simulink library "lib_controller"  (R2015a)
settings: Solver=ode45  StartTime=0.0  StopTime=10.0  RelTol=1e-3
values from neighbouring files (symbols this model uses):
  CG_0 = [0,0,0.02]'    [SetupComplete.m]
  g = 9.81    [SetupComplete.m]
  h_M = 0.064    [SetupComplete.m]
  I_BAC_0 = [ Ix,0,Ixz;0,Iy,0;Ixz,0,Iz]    [SetupComplete.m]
  l = 0.3450    (= 0.345)    [NDI_components.m]    (also in SetupComplete.m; robust_controller.m)
  m = 3.51    [SetupComplete.m]
  m_0 = 2.61    [SetupComplete.m]
  m_M = 0.300    (= 0.3)    [SetupComplete.m]
  T_sim = 0.01    [Run3Copter.m]
undefined symbols (not defined in the file or in its folder): Theta_1_roll_last, Theta_2_roll_last, Theta_3_roll_last, V_long_lastA_w_z, V_long_lastAoA, V_roll_last, V_yaw_last, W_long_lastA_w_z, W_long_lastAoA, W_roll_last, W_yaw_last
libraries: simulink x65, Adaptive_FaultTolerantControl x8, lib_controller x5, qcatlib x4, dspinverses x4, aerolibtransform2 x3, aerolib6dofsys x1
(part 3 of 10)

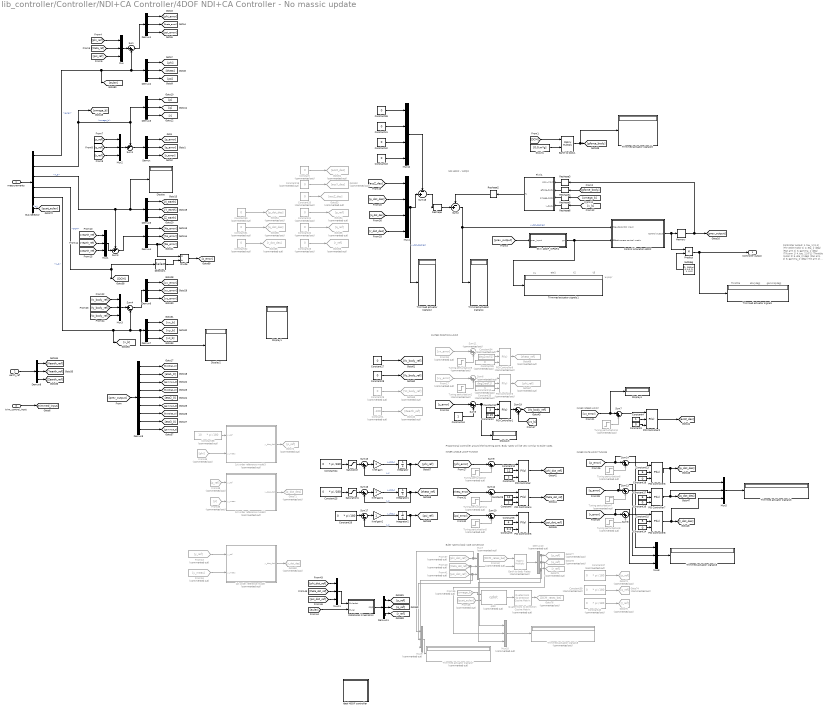
== system lib_controller/Controller/NDI+CA Controller/4DOF NDI+CA Controller - No massic update ==
  note: w
      | p
      | q
      | r
  note: t1
  note: t2
  note: t3
  note: eta1
  note: OUTER POSITION LOOP
  note: gamma[deg]
  note: eta [deg]
  note: Throttle
  note: Controller output:
      | 1. tau_1 [0-1] (Thr ottle motor 1)
      | 2. eta_1 (deg)  (Pan arm 1)
      | 3. gamma_1 (deg)  (Tilt arm 1)
      |
      | 4. tau_2 [0-1] (Throttle motor 2)
      | 5. eta_2 (deg)  (Pan arm 2)
      | 6. gamma_2 (deg)  (Tilt arm 2)
      |
      | 7. tau_3 [0-1] (Throttle motor 3)
      | 8. eta_3 (deg)  (Pan arm  3)
      | 9. gamma_3 (deg)  (Tilt arm 3)
  note: Proportional controller around the hovering point. Body rates will be very similar to euler rates.
  note: INNER RATE LOOP TUNING
  note: INNER ANGLE LOOP TUNING
  note: INNER SPEED LOOP
  note: NDI 4DOF - WPQR
  note: Euler rate to body rate conversion
  measurements : Inport
  earth_ref : Inport  Port=2
  trim_control_input : Inport  Port=3
  1st order reference model : Subsystem  Commented=on  mask(1st order model reference block){Kref=1, Kb=20, fi=0.25, fc=0.5, Kf=1}
      mask prompts: Kref "1st order reference gain"; Kb "Bandwidth gain"; fi "Integral gain"; fc "Command FF gain"; Kf "Command_dot FF gain"
      mask help:
      | Generates a desired first order derivative of a commanded output taking
      | into account the current measured output.
      | Kref is the gain that determines the first order system between y_ref and
      | y_commanded signals. Ycom/Yref = Kref/(1 + Kref)
      | fi and fc can be defaulted to 0.25 and 0.5 for a critically damped 2nd
      | order response between y_meas and the error signal (y_com - y_meas) considering
      | a perfect dynamic inversion.
      mask Help:
      | Juan Herrero Macias <jn.herrerom@gmail.com>
      | This architecture can be found and explained in Fault-tolerant Flight
      | Control and Guidance Systems, Ducard, Guillaume.
      mask TypeOptions Kref: Kref gain/Gain
      mask TypeOptions Kb: Bandwidth gain/Gain
      mask TypeOptions fi: Integral gain/Gain
      mask TypeOptions fc: Command FF gain/Gain
      mask TypeOptions Kf: Command_dot FF gain/Gain
  1st order reference model2 : Subsystem  Commented=on  mask(1st order model reference block){Kref=2, Kb=2, fi=0.25, fc=0.5, Kf=1}
      mask prompts: Kref "1st order reference gain"; Kb "Bandwidth gain"; fi "Integral gain"; fc "Command FF gain"; Kf "Command_dot FF gain"
      mask help:
      | Generates a desired first order derivative of a commanded output taking
      | into account the current measured output.
      | Kref is the gain that determines the first order system between y_ref and
      | y_commanded signals. Ycom/Yref = Kref/(1 + Kref)
      | fi and fc can be defaulted to 0.25 and 0.5 for a critically damped 2nd
      | order response between y_meas and the error signal (y_com - y_meas) considering
      | a perfect dynamic inversion.
      mask Help:
      | Juan Herrero Macias <jn.herrerom@gmail.com>
      | This architecture can be found and explained in Fault-tolerant Flight
      | Control and Guidance Systems, Ducard, Guillaume.
      mask TypeOptions Kref: Kref gain/Gain
      mask TypeOptions Kb: Bandwidth gain/Gain
      mask TypeOptions fi: Integral gain/Gain
      mask TypeOptions fc: Command FF gain/Gain
      mask TypeOptions Kf: Command_dot FF gain/Gain
  1st order reference model3 : Subsystem  Commented=on  mask(1st order model reference block){Kref=2, Kb=2, fi=0.25, fc=0, Kf=0}
      mask prompts: Kref "1st order reference gain"; Kb "Bandwidth gain"; fi "Integral gain"; fc "Command FF gain"; Kf "Command_dot FF gain"
      mask help:
      | Generates a desired first order derivative of a commanded output taking
      | into account the current measured output.
      | Kref is the gain that determines the first order system between y_ref and
      | y_commanded signals. Ycom/Yref = Kref/(1 + Kref)
      | fi and fc can be defaulted to 0.25 and 0.5 for a critically damped 2nd
      | order response between y_meas and the error signal (y_com - y_meas) considering
      | a perfect dynamic inversion.
      mask Help:
      | Juan Herrero Macias <jn.herrerom@gmail.com>
      | This architecture can be found and explained in Fault-tolerant Flight
      | Control and Guidance Systems, Ducard, Guillaume.
      mask TypeOptions Kref: Kref gain/Gain
      mask TypeOptions Kb: Bandwidth gain/Gain
      mask TypeOptions fi: Integral gain/Gain
      mask TypeOptions fc: Command FF gain/Gain
      mask TypeOptions Kf: Command_dot FF gain/Gain
  Bus Selector : BusSelector  OutputSignals=euler,omega_b,X_e,DCM,V_b,q
  Constant{,19..23,29..33,35} (12 alike) : Constant  Commented=on  Value=0
  Constant1 : Constant  Commented=on  Value=-100
  Constant10 : Constant  Value=12
  Constant11 : Constant  Value=3
  Constant12 : Constant  Commented=on  Value=deg2rad(1)
  Constant13 : Constant  Value=6
  Constant{3,14,16,18,27..28,36,41..43} (10 alike) : Constant  Value=0
  Constant15 : Constant  Value=5
  Constant17 : Constant  Value=6
  Constant2 : Constant  Value=0.15
  Constant24 : Constant  Value="0     * pi /180"
  Constant25 : Constant  Value="0     * pi /180"
  Constant26 : Constant  Value="0     * pi /180"
  Constant34 : Constant  Commented=on  Value=deg2rad(1)
  Constant37 : Constant  Commented=on  Value="0     * pi /180"
  Constant38 : Constant  Commented=on  Value="10     * pi /180"
  Constant39 : Constant  Commented=on  Value="0     * pi /180"
  Constant4 : Constant
  Constant40 : Constant  Commented=on  Value="0     * pi /180"
  Constant44 : Constant
  Constant5 : Constant  Value=0.4
  Constant6 : Constant  Value=4
  Constant7 : Constant  Value=3
  Constant8 : Constant  Value=12
  Constant9 : Constant  Value=3
  Control Allocation 4DOF : Subsystem  Variant=on  OverrideUsingVariant=(default)
  Demux{,1..8,11} (10 alike) : Demux  Outputs=3
  Demux10 : Demux  Commented=on  Outputs=3
  Demux9 : Demux  Outputs=9
  Display{,1..4} (5 alike) : Display
  Divide : Product  Inputs=*/
  Earth to body Rates : Product  Commented=on  Multiplication=Matrix(*)
  Earth to body1 : Product  Multiplication=Matrix(*)
  F(X)1 : MATLAB Function  TreatAsAtomicUnit=on
  From13 : From  Commented=on  GotoTag=y_ref
  From17 : From  Commented=on  GotoTag=vy_error
  From18 : From  Commented=on  GotoTag=vx_error
  From25 : From  Commented=on  GotoTag=quat_euler
  From34 : From  Commented=on  GotoTag=y_meas
  From35 : From  Commented=on  GotoTag=phi
  From36 : From  Commented=on  GotoTag=omega_b
  From37 : From  Commented=on  GotoTag=phi_dot_ref
  From38 : From  Commented=on  GotoTag=p_ref
  From39 : From  Commented=on  GotoTag=p
  From40 : From  Commented=on  GotoTag=theta_dot_ref
  From41 : From  Commented=on  GotoTag=psi_dot_ref
  From42 : From  Commented=on  GotoTag=DCM_rates_be
  G(X) 4DOF_WPQR1 : MATLAB Function  TreatAsAtomicUnit=on
  Goto40 : Goto  Commented=on  GotoTag=Zearth_ref
  Goto51 : Goto  Commented=on  GotoTag=accX_des
  Goto52 : Goto  Commented=on  GotoTag=accY_des
  Goto53 : Goto  Commented=on  GotoTag=accZ_des
  Goto{54,72..73,77} (4 alike) : Goto  Commented=on  GotoTag=p_ref
  Goto55 : Goto  Commented=on  GotoTag=q_ref
  Goto56 : Goto  Commented=on  GotoTag=r_ref
  Goto60 : Goto  Commented=on  GotoTag=y_dot_des
  Goto63 : Goto  Commented=on  GotoTag=Vz_body_ref
  Goto64 : Goto  Commented=on  GotoTag=p_dot_des
  Goto65 : Goto  Commented=on  GotoTag=q_dot_des
  Goto66 : Goto  Commented=on  GotoTag=r_dot_des
  Goto67 : Goto  Commented=on  GotoTag=phi_ref
  Goto68 : Goto  Commented=on  GotoTag=theta_ref
  Goto71 : Goto  Commented=on  GotoTag=p_dot_des
  Goto74 : Goto  Commented=on  GotoTag=q_ref
  Goto75 : Goto  Commented=on  GotoTag=r_ref
  Goto76 : Goto  Commented=on  GotoTag=DCM_rates_be
  Goto78 : Goto  Commented=on  GotoTag=q_ref
  Goto79 : Goto  Commented=on  GotoTag=r_ref
  Gravity : Constant  Value=[0;0;m*g]
  Ideal 4DOF controller : Subsystem
  Integrator : Integrator
  Integrator1 : Integrator
  Integrator2 : Integrator
  Kref gain : Gain
  Kref gain1 : Gain
  Kref gain2 : Gain
  Memory : Memory  X0=[0,0,0,0,0,0,0,0,0]  LinearizeAsDelay=on
  Mux{,1..3,5,8,11} (7 alike) : Mux  Inputs=3
  Mux10 : Mux  Commented=on  Inputs=3
  Mux12 : Mux
  Mux4 : Mux
  Mux7 : Mux  Commented=on  Inputs=3
  Mux9 : Mux  Commented=on  Inputs=3
  PID Controller{,1..2,4..5,8} (6 alike) : simulink/Continuous/PID Controller  Controller=PI  TimeDomain=Continuous-time  SampleTime=-1  IntegratorMethod=Forward Euler  FilterMethod=Forward Euler  Form=Parallel  UseFilter=on  ControllerParametersSource=external  P=1  I=1  D=0  N=100  InitialConditionSource=internal  InitialConditionForIntegrator=0  InitialConditionForFilter=0  ExternalReset=none  LimitOutput=off  UpperSaturationLimit=inf  LowerSaturationLimit=-inf  LinearizeAsGain=on  AntiWindupMode=none  Kb=1  TrackingMode=off  Kt=1  PParamMin=[]  PParamMax=[]  IParamMin=[]  IParamMax=[]  DParamMin=[]  DParamMax=[]  NParamMin=[]  NParamMax=[]  KbParamMin=[]  KbParamMax=[]  KtParamMin=[]  KtParamMax=[]  POutMin=[]  POutMax=[]  IOutMin=[]  IOutMax=[]  DOutMin=[]  DOutMax=[]  NOutMin=[]  NOutMax=[]  KbOutMin=[]  KbOutMax=[]  KtOutMin=[]  KtOutMax=[]  IntegratorOutMin=[]  IntegratorOutMax=[]  FilterOutMin=[]  FilterOutMax=[]  SumOutMin=[]  SumOutMax=[]  SumI1OutMin=[]  SumI1OutMax=[]  SumI2OutMin=[]  SumI2OutMax=[]  SumI3OutMin=[]  SumI3OutMax=[]  SumDOutMin=[]  SumDOutMax=[]  SaturationOutMin=[]  SaturationOutMax=[]  IntegratorContinuousStateAttributes=''  IntegratorStateMustResolveToSignalObject=off  IntegratorRTWStateStorageClass=Auto  FilterContinuousStateAttributes=''  FilterStateMustResolveToSignalObject=off  FilterRTWStateStorageClass=Auto  DifferentiatorICPrevScaledInput=0  DifferentiatorOutMin=[]  DifferentiatorOutMax=[]
  PID Controller3 : simulink/Continuous/PID Controller  Commented=on  Controller=PI  TimeDomain=Continuous-time  SampleTime=-1  IntegratorMethod=Forward Euler  FilterMethod=Forward Euler  Form=Parallel  UseFilter=on  ControllerParametersSource=external  P=1  I=1  D=0  N=100  InitialConditionSource=internal  InitialConditionForIntegrator=0  InitialConditionForFilter=0  ExternalReset=none  LimitOutput=off  UpperSaturationLimit=inf  LowerSaturationLimit=-inf  LinearizeAsGain=on  AntiWindupMode=none  Kb=1  TrackingMode=off  Kt=1  PParamMin=[]  PParamMax=[]  IParamMin=[]  IParamMax=[]  DParamMin=[]  DParamMax=[]  NParamMin=[]  NParamMax=[]  KbParamMin=[]  KbParamMax=[]  KtParamMin=[]  KtParamMax=[]  POutMin=[]  POutMax=[]  IOutMin=[]  IOutMax=[]  DOutMin=[]  DOutMax=[]  NOutMin=[]  NOutMax=[]  KbOutMin=[]  KbOutMax=[]  KtOutMin=[]  KtOutMax=[]  IntegratorOutMin=[]  IntegratorOutMax=[]  FilterOutMin=[]  FilterOutMax=[]  SumOutMin=[]  SumOutMax=[]  SumI1OutMin=[]  SumI1OutMax=[]  SumI2OutMin=[]  SumI2OutMax=[]  SumI3OutMin=[]  SumI3OutMax=[]  SumDOutMin=[]  SumDOutMax=[]  SaturationOutMin=[]  SaturationOutMax=[]  IntegratorContinuousStateAttributes=''  IntegratorStateMustResolveToSignalObject=off  IntegratorRTWStateStorageClass=Auto  FilterContinuousStateAttributes=''  FilterStateMustResolveToSignalObject=off  FilterRTWStateStorageClass=Auto  DifferentiatorICPrevScaledInput=0  DifferentiatorOutMin=[]  DifferentiatorOutMax=[]
  PID Controller6 : simulink/Continuous/PID Controller  Controller=PI  TimeDomain=Continuous-time  SampleTime=-1  IntegratorMethod=Forward Euler  FilterMethod=Forward Euler  Form=Parallel  UseFilter=on  ControllerParametersSource=external  P=121.80671459326  I=327.532586687046  D=0  N=100  InitialConditionSource=internal  InitialConditionForIntegrator=0  InitialConditionForFilter=0  ExternalReset=none  LimitOutput=off  UpperSaturationLimit=inf  LowerSaturationLimit=-inf  LinearizeAsGain=on  AntiWindupMode=none  Kb=1  TrackingMode=off  Kt=1  PParamMin=[]  PParamMax=[]  IParamMin=[]  IParamMax=[]  DParamMin=[]  DParamMax=[]  NParamMin=[]  NParamMax=[]  KbParamMin=[]  KbParamMax=[]  KtParamMin=[]  KtParamMax=[]  POutMin=[]  POutMax=[]  IOutMin=[]  IOutMax=[]  DOutMin=[]  DOutMax=[]  NOutMin=[]  NOutMax=[]  KbOutMin=[]  KbOutMax=[]  KtOutMin=[]  KtOutMax=[]  IntegratorOutMin=[]  IntegratorOutMax=[]  FilterOutMin=[]  FilterOutMax=[]  SumOutMin=[]  SumOutMax=[]  SumI1OutMin=[]  SumI1OutMax=[]  SumI2OutMin=[]  SumI2OutMax=[]  SumI3OutMin=[]  SumI3OutMax=[]  SumDOutMin=[]  SumDOutMax=[]  SaturationOutMin=[]  SaturationOutMax=[]  IntegratorContinuousStateAttributes=''  IntegratorStateMustResolveToSignalObject=off  IntegratorRTWStateStorageClass=Auto  FilterContinuousStateAttributes=''  FilterStateMustResolveToSignalObject=off  FilterRTWStateStorageClass=Auto  DifferentiatorICPrevScaledInput=0  DifferentiatorOutMin=[]  DifferentiatorOutMax=[]
  PID Controller7 : simulink/Continuous/PID Controller  Controller=PI  TimeDomain=Continuous-time  SampleTime=-1  IntegratorMethod=Forward Euler  FilterMethod=Forward Euler  Form=Parallel  UseFilter=on  ControllerParametersSource=external  P=244.169484479421  I=1759.80724182952  D=0  N=100  InitialConditionSource=internal  InitialConditionForIntegrator=0  InitialConditionForFilter=0  ExternalReset=none  LimitOutput=off  UpperSaturationLimit=inf  LowerSaturationLimit=-inf  LinearizeAsGain=on  AntiWindupMode=none  Kb=1  TrackingMode=off  Kt=1  PParamMin=[]  PParamMax=[]  IParamMin=[]  IParamMax=[]  DParamMin=[]  DParamMax=[]  NParamMin=[]  NParamMax=[]  KbParamMin=[]  KbParamMax=[]  KtParamMin=[]  KtParamMax=[]  POutMin=[]  POutMax=[]  IOutMin=[]  IOutMax=[]  DOutMin=[]  DOutMax=[]  NOutMin=[]  NOutMax=[]  KbOutMin=[]  KbOutMax=[]  KtOutMin=[]  KtOutMax=[]  IntegratorOutMin=[]  IntegratorOutMax=[]  FilterOutMin=[]  FilterOutMax=[]  SumOutMin=[]  SumOutMax=[]  SumI1OutMin=[]  SumI1OutMax=[]  SumI2OutMin=[]  SumI2OutMax=[]  SumI3OutMin=[]  SumI3OutMax=[]  SumDOutMin=[]  SumDOutMax=[]  SaturationOutMin=[]  SaturationOutMax=[]  IntegratorContinuousStateAttributes=''  IntegratorStateMustResolveToSignalObject=off  IntegratorRTWStateStorageClass=Auto  FilterContinuousStateAttributes=''  FilterStateMustResolveToSignalObject=off  FilterRTWStateStorageClass=Auto  DifferentiatorICPrevScaledInput=0  DifferentiatorOutMin=[]  DifferentiatorOutMax=[]
  PID Controller9 : simulink/Continuous/PID Controller  Commented=on  Controller=PI  TimeDomain=Continuous-time  SampleTime=-1  IntegratorMethod=Forward Euler  FilterMethod=Forward Euler  Form=Parallel  UseFilter=on  ControllerParametersSource=external  P=1  I=1  D=0  N=100  InitialConditionSource=internal  InitialConditionForIntegrator=0  InitialConditionForFilter=0  ExternalReset=none  LimitOutput=off  UpperSaturationLimit=inf  LowerSaturationLimit=-inf  LinearizeAsGain=on  AntiWindupMode=none  Kb=1  TrackingMode=off  Kt=1  PParamMin=[]  PParamMax=[]  IParamMin=[]  IParamMax=[]  DParamMin=[]  DParamMax=[]  NParamMin=[]  NParamMax=[]  KbParamMin=[]  KbParamMax=[]  KtParamMin=[]  KtParamMax=[]  POutMin=[]  POutMax=[]  IOutMin=[]  IOutMax=[]  DOutMin=[]  DOutMax=[]  NOutMin=[]  NOutMax=[]  KbOutMin=[]  KbOutMax=[]  KtOutMin=[]  KtOutMax=[]  IntegratorOutMin=[]  IntegratorOutMax=[]  FilterOutMin=[]  FilterOutMax=[]  SumOutMin=[]  SumOutMax=[]  SumI1OutMin=[]  SumI1OutMax=[]  SumI2OutMin=[]  SumI2OutMax=[]  SumI3OutMin=[]  SumI3OutMax=[]  SumDOutMin=[]  SumDOutMax=[]  SaturationOutMin=[]  SaturationOutMax=[]  IntegratorContinuousStateAttributes=''  IntegratorStateMustResolveToSignalObject=off  IntegratorRTWStateStorageClass=Auto  FilterContinuousStateAttributes=''  FilterStateMustResolveToSignalObject=off  FilterRTWStateStorageClass=Auto  DifferentiatorICPrevScaledInput=0  DifferentiatorOutMin=[]  DifferentiatorOutMax=[]
  Product : Product
  Quaternions to Direction Cosine Matrix : aerolibtransform2/Quaternions to  Direction Cosine Matrix  Commented=on
  Reshape : Reshape  OutputDimensionality=Column vector (2-D)
  Reshape2 : Reshape  OutputDimensionality=Column vector (2-D)  OutputDimensions=[6,1]
  Reshape{3..6} (4 alike) : Reshape  OutputDimensions=[6,1]
  Rotational Kinematics : MATLAB Function  TreatAsAtomicUnit=on
  Saturation : Saturate  UpperLimit=30  LowerLimit=-30
  Saturation1 : Saturate  UpperLimit=30  LowerLimit=-30
  Selector1 : Selector  NumberOfDimensions=2  InputPortWidth=[9]  IndexOptions=Index vector (dialog),Index vector (dialog)  Indices=3,3  OutputSizes=1,1
  Sum{,4,15..17} (5 alike) : Sum  Inputs=|+-
  Sum{1..3,18} (4 alike) : Sum  Inputs=-+|
  Sum{5,7..10,12..14,19} (9 alike) : Sum  Inputs=|++
  Sum11 : Sum  Commented=on  Inputs=|++
  Sum6 : Sum  Commented=on  Inputs=|++
  Trimmed actuator signals{,1..6} (7 alike) : Display
  Trimmed actuator signals7 : Display  Commented=on
  Trimmed actuator signals8 : Display  Commented=on
  Tuning perturbation{,5..6,8} (4 alike) : Step  Commented=on  Time=20  After=3*pi/180  SampleTime=0
  Tuning perturbation2 : Step  Commented=on  Time=20  SampleTime=0
  Tuning perturbation3 : Step  Commented=on  Time=20  SampleTime=0
  Tuning perturbation4 : Step  Commented=on  Time=20  After=-3*pi/180  SampleTime=0
  Tuning perturbation7 : Step  Commented=on  Time=20  After=-3*pi/180  SampleTime=0
  Tuning perturbation9 : Step  Commented=on  Time=20  SampleTime=0
  qdot : aerolib6dofsys/DCM & Euler Angles (Quaternion)/qdot  Commented=on
  rad2deg : Constant  Value=[1, 180/pi, 0,1,0, 0, 1, 0,0]
  Controller output : Outport
  wires:
  [vz_b] -> Sum19/2
  Sum19/1 -> [Vz_body_ref]
  PID Controller1/1 -> Sum19/1
  Selector1/1 -> Divide/2
  Demux4/3 -> [Ze_error], Divide/1
  Saturation1/1 -> Sum16/1
  Saturation/1 -> Sum15/1
  Sum18/1 -> Reshape/1
  Mux12/1 -> Sum18/1
  Constant43/1 -> Mux12/4
  Constant42/1 -> Mux12/3
  Constant41/1 -> Mux12/2
  Constant36/1 -> Mux12/1
  Mux11/1 -> Rotational Kinematics/1(Eulerdot)
  [psi_dot_ref] -> Mux11/3
  [theta_dot_ref] -> Mux11/2
  [phi_dot_ref] -> Mux11/1
  Rotational Kinematics/1(PQR) -> Demux11/1
  Demux11/3 -> [r_ref]
  Demux11/2 -> [q_ref]
  Demux11/1 -> [p_ref]
  [euler] -> Rotational Kinematics/2(Euler)
  Mux10/1 -> Trimmed actuator signals8/1
  Demux10/3 -> Mux10/3, Goto79/1
  Demux10/2 -> Goto78/1, Mux10/2
  Demux10/1 -> Goto77/1, Mux10/1
  Mux9/1 -> Trimmed actuator signals7/1
  From41/1 -> Mux7/3, Mux9/3
  From40/1 -> Mux7/2, Mux9/2
  From37/1 -> Mux7/1, Mux9/1
  Quaternions to Direction Cosine Matrix/1 -> Goto76/1
  From25/1 -> qdot/2
  qdot/1 -> Quaternions to Direction Cosine Matrix/1
  From36/1 -> qdot/1
  Earth to body Rates/1 -> Demux10/1
  From42/1 -> Earth to body Rates/1
  Mux7/1 -> Earth to body Rates/2
  Bus Selector/6 -> [quat_euler]  "<q>"
  Divide/1 -> [z_error]
  Constant40/1 -> Goto75/1
  Constant39/1 -> Goto74/1
  Constant37/1 -> Goto73/1
  Constant14/1 -> PID Controller8/3
  Constant18/1 -> PID Controller6/3
  Sum17/1 -> Kref gain2/1
  Kref gain2/1 -> Integrator2/1  "y_dot_c"
  Integrator2/1 -> [psi_ref], Sum17/2  "y_c"
  Constant26/1 -> Sum17/1
  Sum16/1 -> Kref gain1/1
  Kref gain1/1 -> Integrator1/1  "y_dot_c"
  Integrator1/1 -> Sum16/2, [theta_ref]  "y_c"
  Constant25/1 -> Saturation1/1
  Sum15/1 -> Kref gain/1
  Kref gain/1 -> Integrator/1  "y_dot_c"
  Integrator/1 -> [phi_ref], Sum15/2  "y_c"
  Constant24/1 -> Saturation/1
  Constant38/1 -> 1st order reference model3/1(y_ref)
  1st order reference model3/1(y_des_dot) -> Goto72/1
  From35/1 -> 1st order reference model3/2(y_meas)
  From38/1 -> 1st order reference model2/1(y_ref)
  1st order reference model2/1(y_des_dot) -> Goto71/1
  From39/1 -> 1st order reference model2/2(y_meas)
  G(X) 4DOF_WPQR1/1(gx) -> Control Allocation 4DOF/2(Effectiveness control matrix), Trimmed actuator signals1/1
  PID Controller9/1 -> Goto68/1
  Tuning perturbation9/1 -> Sum11/2
  From18/1 -> Sum11/1
  Sum11/1 -> PID Controller9/1
  Constant35/1 -> PID Controller9/3
  Constant34/1 -> PID Controller9/2
  PID Controller3/1 -> Goto67/1
  Tuning perturbation2/1 -> Sum6/2
  From17/1 -> Sum6/1
  Sum6/1 -> PID Controller3/1
  Constant33/1 -> PID Controller3/3
  Constant12/1 -> PID Controller3/2
  Constant44/1 -> Sum5/2
  [z_error] -> Sum5/1
  Sum5/1 -> PID Controller1/1, Display3/1
  Constant2/1 -> PID Controller1/3
  Constant11/1 -> PID Controller1/2
  Constant1/1 -> Goto40/1
  [r_dot_des] -> Mux4/4
  [q_dot_des] -> Mux4/3
  [p_dot_des] -> Mux4/2
  [accZ_des] -> Mux4/1
  [prev_output] -> G(X) 4DOF_WPQR1/1(prev_input)
  Control Allocation 4DOF/1(Control output) -> Memory/1, Product/1
  Sum2/1 -> Control Allocation 4DOF/1(Pseudocontrol input), Trimmed actuator signals4/1  "y_dot_desired"
  Constant13/1 -> PID Controller6/2
  Sum3/1 -> Demux4/1
  Constant32/1 -> Goto66/1
  Constant31/1 -> Goto65/1
  Constant30/1 -> Goto64/1
  Memory/1 -> [prev_output], Reshape3/1
  [DCM] -> Earth to body1/1
  Mux8/1 -> Trimmed actuator signals5/1
  [r_error] -> Sum8/1, Mux8/3
  [q_error] -> Sum13/1, Mux8/2
  [p_error] -> Sum14/1, Mux8/1
  [psi_error] -> Sum10/1
  [theta_error] -> Sum12/1
  [phi_error] -> Sum9/1
  Constant29/1 -> Goto63/1
  Constant28/1 -> [Vy_body_ref]
  Constant27/1 -> [Vx_body_ref]
  PID Controller2/1 -> [accZ_des]
  Mux5/1 -> Trimmed actuator signals3/1
  1st order reference model/1(y_des_dot) -> Goto60/1
  From34/1 -> 1st order reference model/2(y_meas)
  From13/1 -> 1st order reference model/1(y_ref)
  rad2deg/1 -> Product/2
  Product/1 -> Controller output/1, Trimmed actuator signals/1
  Constant23/1 -> Goto56/1
  Constant22/1 -> Goto55/1
  Constant21/1 -> Goto54/1
  Constant20/1 -> Goto53/1
  Constant19/1 -> Goto52/1
  Constant/1 -> Goto51/1
  [v_b] -> Reshape6/1
  Reshape6/1 -> F(X)1/4(v_body)
  Reshape5/1 -> F(X)1/3(omega_body)
  Reshape4/1 -> F(X)1/2(gforce_body)
  [omega_b] -> Reshape5/1
  Reshape3/1 -> F(X)1/1(prev_input)
  Reshape2/1 -> Sum2/1
  Reshape/1 -> Sum2/2
  Mux4/1 -> Sum18/2, Trimmed actuator signals2/1  "y_dot_desired"
  Tuning perturbation7/1 -> Sum13/2
  Tuning perturbation6/1 -> Sum14/2
  Tuning perturbation8/1 -> Sum8/2
  Sum13/1 -> PID Controller7/1
  Sum8/1 -> PID Controller8/1
  Sum14/1 -> PID Controller6/1
  Constant16/1 -> PID Controller7/3
  Constant17/1 -> PID Controller7/2
  Constant15/1 -> PID Controller8/2
  PID Controller8/1 -> [r_dot_des], Mux5/3
  PID Controller7/1 -> [q_dot_des], Mux5/2
  PID Controller6/1 -> [p_dot_des], Mux5/1
  Tuning perturbation4/1 -> Sum12/2
  Tuning perturbation/1 -> Sum9/2
  Tuning perturbation5/1 -> Sum10/2
  Sum12/1 -> PID Controller4/1
  Sum10/1 -> PID Controller5/1
  Sum9/1 -> PID Controller/1
  Constant7/1 -> PID Controller4/3
  Constant9/1 -> PID Controller/3
  Constant10/1 -> PID Controller/2
  Constant8/1 -> PID Controller4/2
  Constant5/1 -> PID Controller5/3
  Constant6/1 -> PID Controller5/2
  PID Controller5/1 -> [psi_dot_ref]
  PID Controller4/1 -> [theta_dot_ref]
  PID Controller/1 -> [phi_dot_ref]
  Tuning perturbation3/1 -> Sum7/2
  [vz_error] -> Sum7/1, Display4/1
  Sum7/1 -> PID Controller2/1
  Constant3/1 -> PID Controller2/3
  Constant4/1 -> PID Controller2/2
  [gforce_body] -> Reshape4/1
  Earth to body1/1 -> [gforce_body], Trimmed actuator signals6/1
  Gravity/1 -> Earth to body1/2
  F(X)1/1(fx) -> Reshape2/1
  Mux/1 -> Sum/1
  Demux3/3 -> [r]
  Demux3/2 -> [q]
  Demux3/1 -> [p]
  Demux2/1 -> [phi]
  Demux2/2 -> [theta]
  Demux2/3 -> [psi]
  measurements/1 -> Bus Selector/1
  Bus Selector/1 -> Demux2/1, Sum/2, [euler]  "<euler>"
  Bus Selector/2 -> Demux3/1, Sum1/1, [omega_b]  "<omega_b>"
  Sum1/1 -> Demux/1
  Sum/1 -> Demux1/1
  Demux/3 -> [r_error]
  Demux/2 -> [q_error]
  Demux/1 -> [p_error]
  Demux1/1 -> [phi_error]
  Demux1/2 -> [theta_error]
  Demux1/3 -> [psi_error]
  trim_control_input/1 -> [trimmed_input]
  [theta_ref] -> Mux/2
  [phi_ref] -> Mux/1
  [psi_ref] -> Mux/3
  Mux2/1 -> Sum1/2
  [q_ref] -> Mux2/2
  [p_ref] -> Mux2/1
  [r_ref] -> Mux2/3
  Bus Selector/3 -> Sum3/1, Demux5/1, Display/1  "<X_e>"
  Demux5/3 -> [Z_earth]
  Demux5/2 -> [Y_earth]
  Demux5/1 -> [X_earth]
  Demux4/2 -> [Ye_error]
  Demux4/1 -> [Xe_error]
  Mux1/1 -> Sum3/2
  [Yearth_ref] -> Mux1/2
  [Xearth_ref] -> Mux1/1
  [Zearth_ref] -> Mux1/3
  Mux3/1 -> Sum4/1
  Demux7/1 -> [vx_b]
  Demux7/2 -> [vy_b]
  Demux7/3 -> [vz_b]
  Bus Selector/5 -> Demux7/1, Display2/1, Sum4/2, [v_b]  "<V_b>"
  Sum4/1 -> Demux6/1
  Demux6/1 -> [vx_error]
  Demux6/2 -> [vy_error]
  Demux6/3 -> [vz_error]
  [Vy_body_ref] -> Mux3/2
  [Vx_body_ref] -> Mux3/1
  [Vz_body_ref] -> Mux3/3
  Bus Selector/4 -> Selector1/1, [DCM]  "<DCM>"
  Demux8/3 -> [Zearth_ref]
  Demux8/2 -> [Yearth_ref]
  Demux8/1 -> [Xearth_ref]
  earth_ref/1 -> Demux8/1
  [prev_output] -> Demux9/1
  Demux9/1 -> [throttle1_0]
  Demux9/2 -> [eta1_0]
  Demux9/3 -> [gamma1_0]
  Demux9/4 -> [throttle2_0]
  Demux9/5 -> [eta2_0]
  Demux9/6 -> [gamma2_0]
  Demux9/7 -> [throttle3_0]
  Demux9/8 -> [eta3_0]
  Demux9/9 -> [gamma3_0]

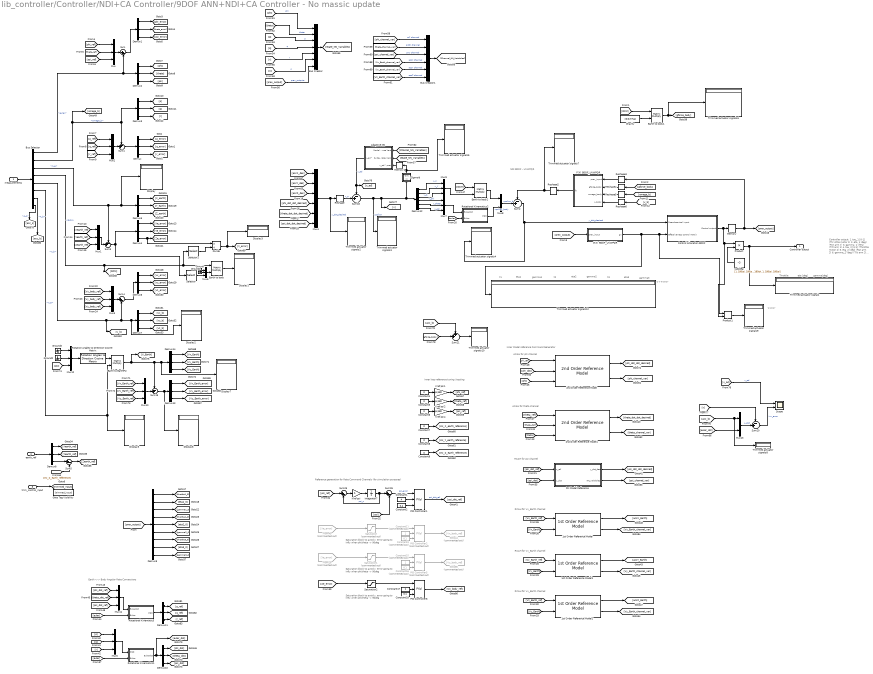
== system lib_controller/Controller/NDI+CA Controller/9DOF ANN+NDI+CA Controller - No massic update ==
  note: Saturation block to avoid z_error going to
      |  infty when phi/theta -> 90deg
  note: Saturation block to avoid z_error going to
      |  infty when phi/theta -> 90deg
  note: RCAH for Vx_Earth channel
  note: RCAH for Vx_Earth channel
  note: RCAH for Vx_Earth channel
  note: gamma3
  note: gamma2
  note: gamma1
  note: eta3
  note: eta2
  note: eta1
  note: t3
  note: t2
  note: t1
  note: u
      | v
      | w
      | p
      | q
      | r
  note: Saturation block to avoid z_error going to
      |  infty when phi/theta -> 90deg
  note: Inner loop reference tuning / testing
  note: Earth <-> Body Angular Rate Conversions
  note: Reference generation for Rate Command Channels (for simulation purposes)
  note: ACAH for phi channel
  note: NDI 9DOF - UVWPQR
  note: Controller output:
      | 1. tau_1 [0-1] (Thr ottle motor 1)
      | 2. eta_1 (deg)  (Pan arm 1)
      | 3. gamma_1 (deg)  (Tilt arm 1)
      |
      | 4. tau_2 [0-1] (Throttle motor 2)
      | 5. eta_2 (deg)  (Pan arm 2)
      | 6. gamma_2 (deg)  (Tilt arm 2)
      |
      | 7. tau_3 [0-1] (Throttle motor 3)
      | 8. eta_3 (deg)  (Pan arm  3)
      | 9. gamma_3 (deg)  (Tilt arm 3)
  note: Throttle
  note: eta [deg]
  note: gamma[deg]
  note: ACAH for theta channel
  note: RCAH for psi channel
  note: Inner Model reference Command Generator
  note: w
      | p
      | q
      | r
  measurements : Inport
  earth_ref : Inport  Port=2
  trim_control_input : Inport  Port=3
  1st Order Reference Model : lib_controller/1st Order Reference Model  tau=0.25  r=1
  1st Order Reference Model1 : lib_controller/1st Order Reference Model  tau=0.25  r=1
  1st Order Reference Model2 : lib_controller/1st Order Reference Model  tau=0.25  r=1
  2nd Order Reference Model : lib_controller/2nd Order Reference Model  omega_n=4  xi=1.1  r=0
  2nd Order Reference Model1 : lib_controller/2nd Order Reference Model  omega_n=4  xi=1.1  r=0
  Adaptive NN : Subsystem  Variant=on  VariantControl=Variant  OverrideUsingVariant=NN on AoA
      mask Display:
      | image(imread('ANN.png'))
      | 
      | 
      | port_label('input', 2, 'State vars')
      | port_label('input', 1, 'Channel vars')
      | port_label('input', 3, 'v prev')
      | 
      | port_label('output', 1, 'v_ad^')
  Bus Creator : BusCreator  Inputs=7
  Bus Creator1 : BusCreator  Inputs=6
  Bus Selector : BusSelector  OutputSignals=euler,omega_b,X_e,DCM,V_b,V_e,A_b,A_s
  Constant1 : Constant  Value=4
  Constant11 : Constant  Commented=on
  Constant15 : Constant  Commented=on
  Constant16 : Constant  Commented=on  Value=0.1
  Constant17 : Constant
  Constant18 : Constant  Value=0.1
  Constant2 : Constant  Value=0.4
  Constant3 : Constant  Commented=on  Value=0.1
  Constant{4..9} (6 alike) : Constant  Value=0
  Control Allocation 9DOF : Subsystem  Variant=on  OverrideUsingVariant=(default)
  Demux{,1..8,10..11,13..14} (13 alike) : Demux  Outputs=3
  Demux12 : Demux  Outputs=6
  Demux9 : Demux  Outputs=9
  Display{,1..3,5..7} (7 alike) : Display
  Divide : Product  Inputs=*/
  Earth to EarthPsi : Product  Multiplication=Matrix(*)
  Earth to body : Product  Multiplication=Matrix(*)
  Earth to body1 : Product  Multiplication=Matrix(*)
  Earth to body2 : Product  Multiplication=Matrix(*)
  F(X) 9DOF_UVWPQR : MATLAB Function  TreatAsAtomicUnit=on
  From28 : From  Commented=on  GotoTag=Ye_error
  From49 : From  Commented=on  GotoTag=Xe_error
  G(X) 9DOF_UVWPQR : MATLAB Function  TreatAsAtomicUnit=on
  Goto Tag Visibility : GotoTagVisibility  GotoTag=trimmed_input
  Goto44 : Goto  Commented=on  GotoTag=Vx_body_ref
  Goto85 : Goto  Commented=on  GotoTag=Vy_body_ref
  Gravity : Constant  Value=[0;0;m*g]
  Ground{,1..3} (4 alike) : Ground
  Integrator7 : Integrator
  Kref psi : Gain
  Kref psi1 : Gain  Gain=pi/180
  Kref psi2 : Gain  Gain=pi/180
  Kref psi4 : Gain  Gain=pi/180
  Memory : Memory  X0=[0,0,0,0,0,0,0,0,0]  LinearizeAsDelay=on
  Memory1 : Memory
  Mux{,1..3,5..7,9..12} (11 alike) : Mux  Inputs=3
  Mux13 : Mux  Inputs=2
  Mux4 : Mux  Inputs=6
  Mux8 : Mux  Inputs=2
  PID Controller1 : simulink/Continuous/PID Controller  Controller=PI  TimeDomain=Continuous-time  SampleTime=-1  IntegratorMethod=Forward Euler  FilterMethod=Forward Euler  Form=Parallel  UseFilter=on  ControllerParametersSource=external  P=1  I=1  D=0  N=100  InitialConditionSource=internal  InitialConditionForIntegrator=0  InitialConditionForFilter=0  ExternalReset=none  LimitOutput=off  UpperSaturationLimit=inf  LowerSaturationLimit=-inf  LinearizeAsGain=on  AntiWindupMode=none  Kb=1  TrackingMode=off  Kt=1  PParamMin=[]  PParamMax=[]  IParamMin=[]  IParamMax=[]  DParamMin=[]  DParamMax=[]  NParamMin=[]  NParamMax=[]  KbParamMin=[]  KbParamMax=[]  KtParamMin=[]  KtParamMax=[]  POutMin=[]  POutMax=[]  IOutMin=[]  IOutMax=[]  DOutMin=[]  DOutMax=[]  NOutMin=[]  NOutMax=[]  KbOutMin=[]  KbOutMax=[]  KtOutMin=[]  KtOutMax=[]  IntegratorOutMin=[]  IntegratorOutMax=[]  FilterOutMin=[]  FilterOutMax=[]  SumOutMin=[]  SumOutMax=[]  SumI1OutMin=[]  SumI1OutMax=[]  SumI2OutMin=[]  SumI2OutMax=[]  SumI3OutMin=[]  SumI3OutMax=[]  SumDOutMin=[]  SumDOutMax=[]  SaturationOutMin=[]  SaturationOutMax=[]  IntegratorContinuousStateAttributes=''  IntegratorStateMustResolveToSignalObject=off  IntegratorRTWStateStorageClass=Auto  FilterContinuousStateAttributes=''  FilterStateMustResolveToSignalObject=off  FilterRTWStateStorageClass=Auto  DifferentiatorICPrevScaledInput=0  DifferentiatorOutMin=[]  DifferentiatorOutMax=[]
  PID Controller2 : simulink/Continuous/PID Controller  Commented=on  Controller=PI  TimeDomain=Continuous-time  SampleTime=-1  IntegratorMethod=Forward Euler  FilterMethod=Forward Euler  Form=Parallel  UseFilter=on  ControllerParametersSource=external  P=1  I=1  D=0  N=100  InitialConditionSource=internal  InitialConditionForIntegrator=0  InitialConditionForFilter=0  ExternalReset=none  LimitOutput=off  UpperSaturationLimit=inf  LowerSaturationLimit=-inf  LinearizeAsGain=on  AntiWindupMode=none  Kb=1  TrackingMode=off  Kt=1  PParamMin=[]  PParamMax=[]  IParamMin=[]  IParamMax=[]  DParamMin=[]  DParamMax=[]  NParamMin=[]  NParamMax=[]  KbParamMin=[]  KbParamMax=[]  KtParamMin=[]  KtParamMax=[]  POutMin=[]  POutMax=[]  IOutMin=[]  IOutMax=[]  DOutMin=[]  DOutMax=[]  NOutMin=[]  NOutMax=[]  KbOutMin=[]  KbOutMax=[]  KtOutMin=[]  KtOutMax=[]  IntegratorOutMin=[]  IntegratorOutMax=[]  FilterOutMin=[]  FilterOutMax=[]  SumOutMin=[]  SumOutMax=[]  SumI1OutMin=[]  SumI1OutMax=[]  SumI2OutMin=[]  SumI2OutMax=[]  SumI3OutMin=[]  SumI3OutMax=[]  SumDOutMin=[]  SumDOutMax=[]  SaturationOutMin=[]  SaturationOutMax=[]  IntegratorContinuousStateAttributes=''  IntegratorStateMustResolveToSignalObject=off  IntegratorRTWStateStorageClass=Auto  FilterContinuousStateAttributes=''  FilterStateMustResolveToSignalObject=off  FilterRTWStateStorageClass=Auto  DifferentiatorICPrevScaledInput=0  DifferentiatorOutMin=[]  DifferentiatorOutMax=[]
  PID Controller5 : simulink/Continuous/PID Controller  Commented=on  Controller=PI  TimeDomain=Continuous-time  SampleTime=-1  IntegratorMethod=Forward Euler  FilterMethod=Forward Euler  Form=Parallel  UseFilter=on  ControllerParametersSource=external  P=1  I=1  D=0  N=100  InitialConditionSource=internal  InitialConditionForIntegrator=0  InitialConditionForFilter=0  ExternalReset=none  LimitOutput=off  UpperSaturationLimit=inf  LowerSaturationLimit=-inf  LinearizeAsGain=on  AntiWindupMode=none  Kb=1  TrackingMode=off  Kt=1  PParamMin=[]  PParamMax=[]  IParamMin=[]  IParamMax=[]  DParamMin=[]  DParamMax=[]  NParamMin=[]  NParamMax=[]  KbParamMin=[]  KbParamMax=[]  KtParamMin=[]  KtParamMax=[]  POutMin=[]  POutMax=[]  IOutMin=[]  IOutMax=[]  DOutMin=[]  DOutMax=[]  NOutMin=[]  NOutMax=[]  KbOutMin=[]  KbOutMax=[]  KtOutMin=[]  KtOutMax=[]  IntegratorOutMin=[]  IntegratorOutMax=[]  FilterOutMin=[]  FilterOutMax=[]  SumOutMin=[]  SumOutMax=[]  SumI1OutMin=[]  SumI1OutMax=[]  SumI2OutMin=[]  SumI2OutMax=[]  SumI3OutMin=[]  SumI3OutMax=[]  SumDOutMin=[]  SumDOutMax=[]  SaturationOutMin=[]  SaturationOutMax=[]  IntegratorContinuousStateAttributes=''  IntegratorStateMustResolveToSignalObject=off  IntegratorRTWStateStorageClass=Auto  FilterContinuousStateAttributes=''  FilterStateMustResolveToSignalObject=off  FilterRTWStateStorageClass=Auto  DifferentiatorICPrevScaledInput=0  DifferentiatorOutMin=[]  DifferentiatorOutMax=[]
  PID Controller6 : simulink/Continuous/PID Controller  Controller=PI  TimeDomain=Continuous-time  SampleTime=-1  IntegratorMethod=Forward Euler  FilterMethod=Forward Euler  Form=Parallel  UseFilter=on  ControllerParametersSource=external  P=1  I=1  D=0  N=100  InitialConditionSource=internal  InitialConditionForIntegrator=0  InitialConditionForFilter=0  ExternalReset=none  LimitOutput=off  UpperSaturationLimit=inf  LowerSaturationLimit=-inf  LinearizeAsGain=on  AntiWindupMode=none  Kb=1  TrackingMode=off  Kt=1  PParamMin=[]  PParamMax=[]  IParamMin=[]  IParamMax=[]  DParamMin=[]  DParamMax=[]  NParamMin=[]  NParamMax=[]  KbParamMin=[]  KbParamMax=[]  KtParamMin=[]  KtParamMax=[]  POutMin=[]  POutMax=[]  IOutMin=[]  IOutMax=[]  DOutMin=[]  DOutMax=[]  NOutMin=[]  NOutMax=[]  KbOutMin=[]  KbOutMax=[]  KtOutMin=[]  KtOutMax=[]  IntegratorOutMin=[]  IntegratorOutMax=[]  FilterOutMin=[]  FilterOutMax=[]  SumOutMin=[]  SumOutMax=[]  SumI1OutMin=[]  SumI1OutMax=[]  SumI2OutMin=[]  SumI2OutMax=[]  SumI3OutMin=[]  SumI3OutMax=[]  SumDOutMin=[]  SumDOutMax=[]  SaturationOutMin=[]  SaturationOutMax=[]  IntegratorContinuousStateAttributes=''  IntegratorStateMustResolveToSignalObject=off  IntegratorRTWStateStorageClass=Auto  FilterContinuousStateAttributes=''  FilterStateMustResolveToSignalObject=off  FilterRTWStateStorageClass=Auto  DifferentiatorICPrevScaledInput=0  DifferentiatorOutMin=[]  DifferentiatorOutMax=[]
  Product : Product
  Product1 : Product  Multiplication=Matrix(*)
  Psi Model Reference : Subsystem  mask{tau=0.30, r=1}
      mask prompts: tau "Time Constant"; r "NN Error dynamic ratio"
      mask help:
      | 1st Order Model Reference System
      | Tau is the time constant and sets the dynamics of the reference model.
      | Error dynamic ratio sets how faster compared to the reference model is the
      | NN output going to try to compensate for the inversion error.
      mask Display:
      | K_ref=1/tau;
      | TF = tf([K_ref],[1 K_ref]);
      | 
      | [y,t]=step(TF);
      | S = stepinfo(y,t);
      | 
      | pos = get_param(gcb, 'Position');
      | width = pos(3) - pos(1);
      | height = pos(4) - pos(2);
      | t = t.*width/max(t);
      | y=y.*height/max(y);
      | plot(t,y);
      | S2 = stepinfo(y,t);
      | 
      | if S.Overshoot==0 % 1st order response
      |     text(S2.RiseTime ,height*0.85,['Rise time = ',num2str(S.RiseTime),'s' ]);
      |     text(S2.RiseTime ,height*0.75,['Settling Time = ',num2str(S.SettlingTime)]);
      | 
      | elseif S.Overshoot<0.05 % 2nd order response
      |     text(width*0.5 ,height*0.9,['Rise time = ',num2str(S.RiseTime),'s' ]);
      |     text(width*0.5 ,height*0.8,['Pike time = ',num2str(S.PeakTime),'s' ]);
      |     text(width*0.5 ,height*0.7,['Os = ',num2str(S.Peak)]);
      |     text(width*0.5 ,height*0.6,['SettlingTime = ',num2str(S.SettlingTime)]);
      | else % 2nd order response
      |     text(S2.PeakTime ,S2.Peak*0.85,['Peak time = ',num2str(S.PeakTime),'s' ]);
      |     text(S2.PeakTime ,S2.Peak*0.75,['Os = ',num2str(S.Peak)]);
      |     text(S2.PeakTime ,S2.Peak*0.65,['SettlingTime = ',num2str(S.SettlingTime)]);
      | end
      | 
      | 
      | [num,den] = tfdata(TF);
      | dpoly(num{:},den{:}, 's');
  Reshape : Reshape
  Reshape2 : Reshape  OutputDimensionality=Column vector (2-D)  OutputDimensions=[6,1]
  Reshape{3..6} (4 alike) : Reshape  OutputDimensions=[6,1]
  Rotation Angles to Direction Cosine Matrix : aerolibtransform2/Rotation Angles to Direction Cosine Matrix  rotationOrder=ZYX
  Rotational Kinematics : MATLAB Function  TreatAsAtomicUnit=on
  Rotational Kinematics1 : MATLAB Function  TreatAsAtomicUnit=on
  Rotational Kinematics2 : MATLAB Function  TreatAsAtomicUnit=on
  Saturation : Saturate  Commented=on  UpperLimit=4  LowerLimit=-4
  Saturation1 : Saturate  Commented=on  UpperLimit=4  LowerLimit=-4
  Saturation2 : Saturate  UpperLimit=4  LowerLimit=-4
  Scope : Scope  NumInputPorts=2
      settings: ShowLegends=on  YMin=-4~-10  YMax=1~15  SaveName=ScopeData5
  Selector : Selector  InputPortWidth=3  Indices=[3]
  Selector1 : Selector  NumberOfDimensions=2  InputPortWidth=[9]  IndexOptions=Index vector (dialog),Index vector (dialog)  Indices=3,3  OutputSizes=1,1
  "Sigmoid " : Subsystem  mask{a=0.15}
      mask prompts: a "Sigmoid a param"
      mask TypeOptions a: a/Value
      mask Display:
      | x=-25:0.1:25;
      | 
      | y=(2.0 ./ (1.0 + exp(-a.*x))-1) ;
      | y2=zeros(size(x));
      | 
      | plot(x,y,x,y2);
      | 
      | %text(-20,0.5, ['a= ',num2str(a)])
  Sum{,4..5,25..26} (5 alike) : Sum  Inputs=|+-
  Sum{1..3,18..20} (6 alike) : Sum  Inputs=-+|
  Sum21 : Sum  Inputs=++|
  Trimmed actuator signals{,2..10,12} (11 alike) : Display
  rad2deg : Constant  Value=[1, 180/pi, 180/pi,1, 180/pi, 180/pi, 1, 180/pi, 180/pi]
  Controller output : Outport
  tag scope: trimmed_input=scoped
  wires:
  [Vx_Earth_channel_var] -> Bus Creator1/4  "accX channel"
  [Vy_Earth_channel_var] -> Bus Creator1/5  "accY channel"
  [Vz_Earth_channel_var] -> Bus Creator1/6  "accZ channel"
  [accX_des] -> Mux4/1
  [accY_des] -> Mux4/2
  [accZ_des] -> Mux4/3
  [phi_dot_dot_desired] -> Mux4/4
  [theta_dot_dot_desired] -> Mux4/5
  [psi_dot_dot_desired] -> Mux4/6
  Demux12/2 -> Mux9/2  "v_Y"
  Demux12/3 -> Mux9/3  "v_Z"
  Demux12/1 -> Mux9/1  "v_X"
  Earth to body2/1 -> Mux8/1
  Demux12/4 -> Mux7/1  "v_phi"
  Demux12/5 -> Mux7/2  "v_theta"
  Demux12/6 -> Mux7/3  "v_psi"
  Mux9/1 -> Earth to body2/2
  [DCM] -> Earth to body2/1
  Constant9/1 -> [Inc_Z_earth_reference]
  Constant8/1 -> [Inc_Y_earth_reference]
  Constant17/1 -> PID Controller6/2
  Constant18/1 -> PID Controller6/3
  [Ze_error] -> Saturation2/1
  PID Controller6/1 -> [Vz_body_ref]
  Saturation2/1 -> PID Controller6/1
  Constant15/1 -> PID Controller5/2
  Constant16/1 -> PID Controller5/3
  From28/1 -> Saturation1/1
  PID Controller5/1 -> Goto85/1
  Saturation1/1 -> PID Controller5/1
  1st Order Reference Model2/1 -> [accZ_Earth]
  [Vz_Earth_ref] -> 1st Order Reference Model2/1
  [Vz_Earth] -> 1st Order Reference Model2/2
  1st Order Reference Model2/2 -> [Vz_Earth_channel_var]
  1st Order Reference Model1/1 -> [accY_Earth]
  [Vy_Earth_ref] -> 1st Order Reference Model1/1
  [Vy_Earth] -> 1st Order Reference Model1/2
  1st Order Reference Model1/2 -> [Vy_Earth_channel_var]
  1st Order Reference Model/1 -> [accX_Earth]
  [Vx_Earth_ref] -> 1st Order Reference Model/1
  [Vx_Earth] -> 1st Order Reference Model/2
  1st Order Reference Model/2 -> [Vx_Earth_channel_var]
  Demux9/9 -> [gamma3_0]
  Demux9/8 -> [eta3_0]
  Demux9/7 -> [throttle3_0]
  Demux9/6 -> [gamma2_0]
  Demux9/5 -> [eta2_0]
  Demux9/4 -> [throttle2_0]
  Demux9/3 -> [gamma1_0]
  Demux9/2 -> [eta1_0]
  Demux9/1 -> [throttle1_0]
  [prev_output] -> Demux9/1
  earth_ref/1 -> Demux8/1
  Demux8/1 -> [Xearth_ref]
  Demux8/2 -> [Yearth_ref]
  Bus Selector/4 -> Earth to body/1, Selector1/1, [DCM]  "<DCM>"
  [Vz_body_ref] -> Mux3/3
  [Vx_body_ref] -> Mux3/1
  [Vy_body_ref] -> Mux3/2
  Demux6/3 -> [vz_error]
  Demux6/2 -> [vy_error]
  Demux6/1 -> [vx_error]
  Sum4/1 -> Demux6/1
  Bus Selector/5 -> [v_b], Sum4/2, Display2/1, Demux7/1  "<V_b>"
  Demux7/3 -> [vz_b]
  Demux7/2 -> [vy_b]
  Demux7/1 -> [vx_b]
  Mux3/1 -> Sum4/1
  [Zearth_ref] -> Mux1/3
  [Xearth_ref] -> Mux1/1
  [Yearth_ref] -> Mux1/2
  Mux1/1 -> Sum3/2
  Demux4/1 -> [Xe_error]
  Demux4/2 -> [Ye_error]
  Demux4/3 -> Divide/1, [Ze_error]
  Demux5/1 -> [X_earth]
  Demux5/2 -> [Y_earth]
  Demux5/3 -> [Z_earth]
  Bus Selector/3 -> Display/1, Demux5/1, Sum3/1  "<X_e>"
  [r_ref] -> Mux2/3
  [p_ref] -> Mux2/1
  [q_ref] -> Mux2/2
  Mux2/1 -> Sum1/2
  [psi_ref] -> Mux/3
  [phi_ref] -> Mux/1
  [theta_ref] -> Mux/2
  trim_control_input/1 -> [trimmed_input]
  Demux1/3 -> [psi_error]
  Demux1/2 -> [theta_error]
  Demux1/1 -> [phi_error]
  Demux/1 -> [p_error]
  Demux/2 -> [q_error]
  Demux/3 -> [r_error]
  Sum/1 -> Demux1/1
  Sum1/1 -> Demux/1
  Bus Selector/2 -> [omega_b], Sum1/1, Demux3/1  "<omega_b>"
  Bus Selector/1 -> Sum/2, Demux2/1  "<euler>"
  measurements/1 -> Bus Selector/1
  Demux2/3 -> [psi]
  Demux2/2 -> [theta]
  Demux2/1 -> [phi]
  Demux3/1 -> [p]
  Demux3/2 -> [q]
  Demux3/3 -> [r]
  Mux/1 -> Sum/1
  F(X) 9DOF_UVWPQR/1(fx) -> Reshape2/1
  Gravity/1 -> Earth to body1/2
  Earth to body1/1 -> Trimmed actuator signals6/1, [gforce_body]
  [gforce_body] -> Reshape4/1
  Mux4/1 -> Trimmed actuator signals2/1, Reshape/1  "y_dot_desired"
  Reshape2/1 -> Sum2/1, Trimmed actuator signals7/1
  Reshape3/1 -> F(X) 9DOF_UVWPQR/1(prev_input)
  [omega_b] -> Reshape5/1
  Reshape4/1 -> F(X) 9DOF_UVWPQR/2(gforce_body)
  Reshape5/1 -> F(X) 9DOF_UVWPQR/3(omega_body)
  Reshape6/1 -> F(X) 9DOF_UVWPQR/4(v_body)
  [v_b] -> Reshape6/1
  Product/1 -> Trimmed actuator signals/1, Controller output/1
  rad2deg/1 -> Product/2
  [DCM] -> Earth to body1/1
  Memory/1 -> Reshape3/1, [prev_output]
  Sum3/1 -> Demux4/1, Selector/1
  Sum2/1 -> Trimmed actuator signals4/1, Control Allocation 9DOF/1(Pseudocontrol input)  "y_dot_desired"
  [prev_output] -> G(X) 9DOF_UVWPQR/1(prev_input)
  G(X) 9DOF_UVWPQR/1(gx) -> Product1/1, Control Allocation 9DOF/2(Effectiveness control matrix), Trimmed actuator signals12/1
  Selector/1 -> Mux6/3
  Ground/1 -> Mux6/1
  Ground1/1 -> Mux6/2
  Mux6/1 -> Earth to body/2
  Earth to body/1 -> Display1/1
  Sum18/1 -> Trimmed actuator signals3/1, Demux12/1, "Sigmoid "/1(In), [v]  "upsilon"
  Reshape/1 -> Sum18/2  "v_o"
  Adaptive NN/1(v_ad^) -> [v_ad], Sum18/1  "v_ad"
  "Sigmoid "/1(Out) -> Trimmed actuator signals5/1, Memory1/1
  Memory1/1 -> Adaptive NN/3(v_ad^ prev)
  [euler] -> Rotational Kinematics/2(Euler)
  Demux11/1 -> [p_ref]
  Demux11/2 -> [q_ref]
  Demux11/3 -> [r_ref]
  Rotational Kinematics/1(PQR) -> Demux11/1
  [phi_dot_ref] -> Mux11/1
  [theta_dot_ref] -> Mux11/2
  [psi_dot_ref] -> Mux11/3
  Mux11/1 -> Rotational Kinematics/1(Eulerdot)
  [euler] -> Rotational Kinematics1/2(Euler)
  Mux5/1 -> Rotational Kinematics1/1(PQR)
  [r] -> Mux5/3
  [p] -> Mux5/1
  [q] -> Mux5/2
  Demux10/1 -> [phi_dot]
  Demux10/2 -> [theta_dot]
  Demux10/3 -> [psi_dot]
  Rotational Kinematics1/1(Eulerdot) -> [euler_dot], Demux10/1
  2nd Order Reference Model1/1 -> [theta_dot_dot_desired]
  Mux7/1 -> Rotational Kinematics2/1(Eulerdot)
  [euler] -> Rotational Kinematics2/2(Euler)
  Mux8/1 -> Sum2/2  "upsilon_b"
  Rotational Kinematics2/1(PQR) -> Mux8/2  "upsilon_body"
  Integrator7/1 -> Sum26/1, Sum25/2  "psi_c"
  Kref psi/1 -> Integrator7/1
  Sum25/1 -> Kref psi/1
  [psi_ref] -> Sum25/1
  [psi] -> Sum26/2
  PID Controller1/1 -> [psi_dot_ref]  "psi_dot_ref"
  Constant1/1 -> PID Controller1/2
  Constant2/1 -> PID Controller1/3
  Sum26/1 -> PID Controller1/1  "psi_error"
  Constant11/1 -> PID Controller2/2
  Constant3/1 -> PID Controller2/3
  From49/1 -> Saturation/1
  Selector1/1 -> Divide/2
  Divide/1 -> Display3/1, [z_error]
  [phi_ref] -> 2nd Order Reference Model/1
  [phi_dot] -> 2nd Order Reference Model/2
  [phi] -> 2nd Order Reference Model/3
  2nd Order Reference Model/1 -> [phi_dot_dot_desired]
  [theta_ref] -> 2nd Order Reference Model1/1
  [theta_dot] -> 2nd Order Reference Model1/2
  [theta] -> 2nd Order Reference Model1/3
  [psi_dot_ref] -> Psi Model Reference/1(u_ref)
  [psi_dot] -> Psi Model Reference/2(y_dot)
  Psi Model Reference/1(y_dot_des) -> [psi_dot_dot_desired]
  2nd Order Reference Model/2 -> [phi_channel_var]
  Psi Model Reference/2(NN_variables) -> [psi_channel_var]
  2nd Order Reference Model1/2 -> [theta_channel_var]
  [p] -> Bus Creator/3  "p"
  [theta] -> Bus Creator/2  "theta"
  [q] -> Bus Creator/4  "q"
  [phi] -> Bus Creator/1  "phi"
  [r] -> Bus Creator/5  "r"
  Bus Creator/1 -> [State_NN_Variables]
  [State_NN_Variables] -> Adaptive NN/2(System State Vars)
  [psi_channel_var] -> Bus Creator1/3  "yaw channel"
  [theta_channel_var] -> Bus Creator1/2  "pitch channel"
  [phi_channel_var] -> Bus Creator1/1  "roll channel"
  Bus Creator1/1 -> [Channel_NN_Variables]
  [Channel_NN_Variables] -> Adaptive NN/1(Model Reference Vars)
  [prev_output] -> Bus Creator/7  "prev_outputs"
  [w] -> Bus Creator/6  "w"
  Constant4/1 -> Kref psi1/1
  Constant5/1 -> Kref psi2/1
  Constant6/1 -> Kref psi4/1
  Kref psi1/1 -> [phi_ref]
  Kref psi2/1 -> [theta_ref]
  Kref psi4/1 -> [psi_ref]
  Demux8/3 -> Sum5/1
  Sum5/1 -> [Zearth_ref]
  Constant7/1 -> [Inc_X_earth_reference]
  [Inc_Z_earth_reference] -> Sum5/2
  PID Controller2/1 -> Goto44/1
  Saturation/1 -> PID Controller2/1
  [Vz_Earth_ref] -> Mux10/3
  [Vx_Earth_ref] -> Mux10/1
  [Vy_Earth_ref] -> Mux10/2
  Demux13/3 -> [Vz_Earth_error]
  Demux13/2 -> [Vy_Earth_error]
  Demux13/1 -> [Vx_Earth_error]
  Sum19/1 -> Display6/1, Demux13/1
  Bus Selector/6 -> Earth to EarthPsi/2, Display5/1  "<V_e>"
  Demux14/3 -> [Vz_Earth]
  Demux14/2 -> [Vy_Earth]
  Demux14/1 -> [Vx_Earth]
  Ground3/1 -> Mux12/1
  Ground2/1 -> Mux12/2
  [psi] -> Mux12/3
  Mux12/1 -> Rotation Angles to Direction Cosine Matrix/1
  Rotation Angles to Direction Cosine Matrix/1 -> Earth to EarthPsi/1
  Mux10/1 -> Sum19/2
  Earth to EarthPsi/1 -> Sum19/1, Display7/1, Demux14/1, [V_Earth]
  Bus Selector/7 -> [acc_b]  "<A_b>"
  [euler_dot] -> Mux13/2
  [v_ad] -> Scope/1  "v_ad"
  Mux13/1 -> Sum20/2  "y_dot"
  [v] -> Sum20/1
  Sum20/1 -> Scope/2  "inv_error"
  [acc_b] -> Trimmed actuator signals8/1, Mux13/1
  Product1/1 -> Trimmed actuator signals9/1
  Control Allocation 9DOF/1(Control output) -> Product/1, Product1/2, Memory/1
  Bus Selector/8 -> [acc_s]  "<A_s>"
  [gforce_body] -> Sum21/2
  [acc_b] -> Sum21/1
  Sum21/1 -> Trimmed actuator signals10/1
